simulink model "jiaodu"  (Simulink 7.9)
settings: Solver=ode45  StartTime=0.0  StopTime=50  MinStep=1e-5  RelTol=1e-3
libraries: fuzblock x1
settings Model: Creator=fangzhen  LastModifiedBy=fangzhen
settings SolverCC: ZeroCrossControl=DisableAll

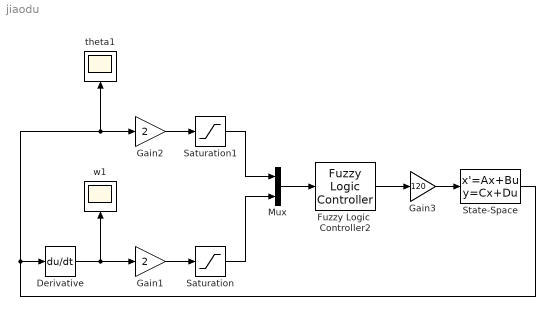
== system jiaodu ==
  Derivative : Derivative
  Fuzzy Logic  Controller2 : fuzblock/Fuzzy Logic  Controller  fis=daolibait
  Gain1 : Gain  Gain=2
  Gain2 : Gain  Gain=2
  Gain3 : Gain  Gain=120
  Mux : Mux  Inputs=2
  Saturation : Saturate  UpperLimit=2  LowerLimit=-2
  Saturation1 : Saturate  UpperLimit=2  LowerLimit=-2
  State-Space : StateSpace  A=[0,1;100/12,0]  B=[0;1/12]  C=[1,0]  D=[0]  X0=[0.2;0]  ContinuousStateAttributes='rad'
  theta1 : Scope
  w1 : Scope
  wires:
  Derivative/1 -> Gain1/1, w1/1
  Gain2/1 -> Saturation1/1
  Gain1/1 -> Saturation/1
  Mux/1 -> Fuzzy Logic  Controller2/1
  Fuzzy Logic  Controller2/1 -> Gain3/1
  Gain3/1 -> State-Space/1
  Saturation/1 -> Mux/2
  Saturation1/1 -> Mux/1
  State-Space/1 -> Derivative/1, Gain2/1, theta1/1
